simulink model "Simulation_with_controller"  (R2014b)
settings: Solver=ode45  StartTime=0.0  StopTime=T  RelTol=1e-3
undefined symbols (not defined in the file): a, L, ref, T, thetainit, Ts, xinit, yinit
settings Model: Creator=Oskar  LastModifiedBy=osklj59
settings OptimizationCC: UseDivisionForNetSlopeComputation=off  SimCompilerOptimization=off
settings DebuggingCC: UnderspecifiedInitializationDetection=Classic  MergeDetectMultiDrivingBlocksExec=none  FrameProcessingCompatibilityMsg=error  StateNameClashWarn=warning
settings RTWCC: RTWCompilerOptimization=off

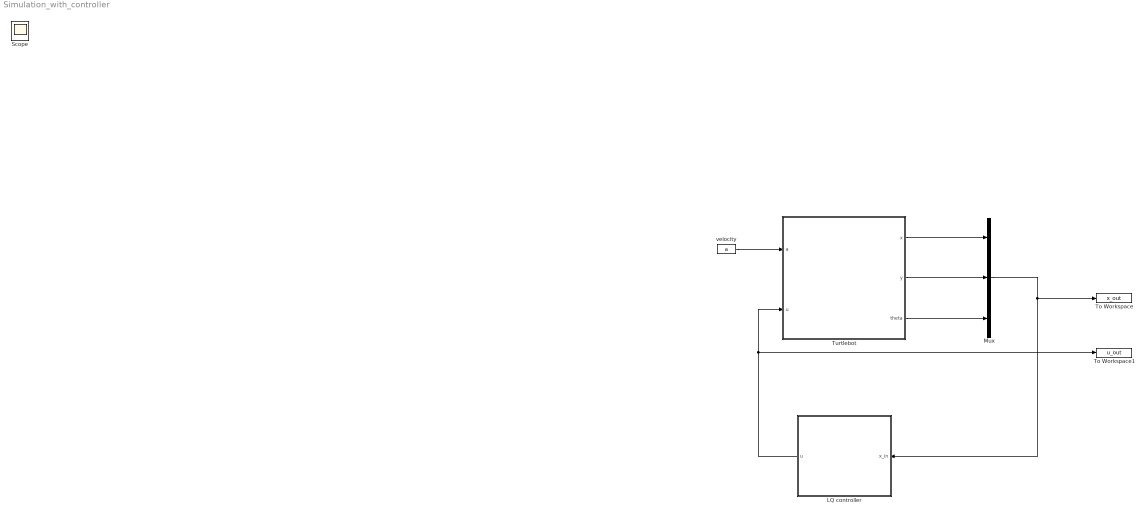
== system Simulation_with_controller ==
  LQ controller : Subsystem
  Mux : Mux  Inputs=3
  To Workspace : ToWorkspace  VariableName=x_out  SaveFormat=Timeseries  SampleTime=-1
  To Workspace1 : ToWorkspace  VariableName=u_out  SaveFormat=Timeseries  SampleTime=-1
  Turtlebot : Subsystem
  velocity : Constant  Value=a
  Scope : Scope
      settings: YMin=-0.4  YMax=0.8
  wires:
  Turtlebot/1("x ") -> Mux/1
  Mux/1 -> To Workspace/1, LQ controller/1(x_in)
  velocity/1 -> Turtlebot/1(a)
  Turtlebot/2("y ") -> Mux/2
  Turtlebot/3("theta ") -> Mux/3
  LQ controller/1(u) -> Turtlebot/2(u), To Workspace1/1

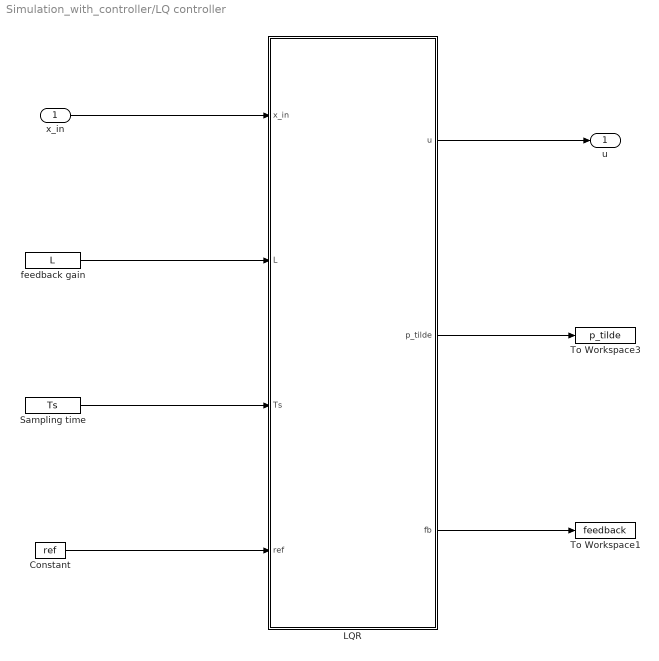
== system Simulation_with_controller/LQ controller ==
  x_in : Inport
  " LQR" : MATLAB Function
  Constant : Constant  Value=ref
  Sampling time : Constant  Value=Ts
  To Workspace1 : ToWorkspace  VariableName=feedback  SaveFormat=Timeseries  SampleTime=-1
  To Workspace3 : ToWorkspace  VariableName=p_tilde  SaveFormat=Timeseries  SampleTime=-1
  feedback gain : Constant  Value=L
  u : Outport
  wires:
  x_in/1 -> " LQR"/1(x_in)
  " LQR"/2(p_tilde) -> To Workspace3/1
  feedback gain/1 -> " LQR"/2(L)
  " LQR"/1(u) -> u/1
  Sampling time/1 -> " LQR"/3(Ts)
  Constant/1 -> " LQR"/4(ref)
  " LQR"/3(fb) -> To Workspace1/1

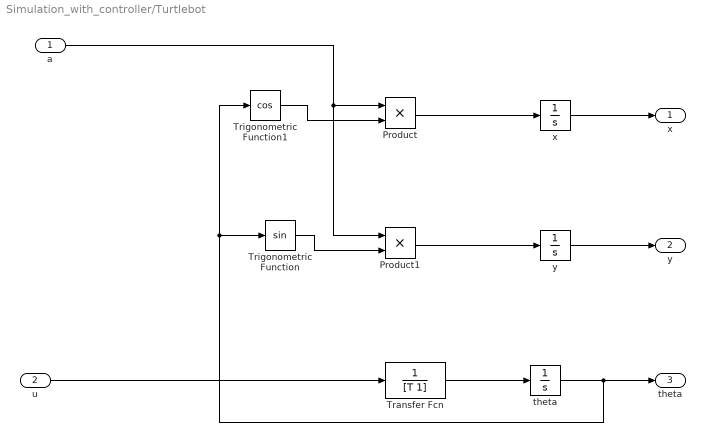
== system Simulation_with_controller/Turtlebot ==
  a : Inport
  u : Inport  Port=2
  Product : Product
  Product1 : Product
  Transfer Fcn : TransferFcn  Denominator=[T 1]
  Trigonometric Function : Trigonometry
  Trigonometric Function1 : Trigonometry  Operator=cos
  theta : Integrator  InitialCondition=thetainit
  x : Integrator  InitialCondition=xinit
  y : Integrator  InitialCondition=yinit
  "x " : Outport  PortDimensions=1
  "y " : Outport  Port=2
  "theta " : Outport  Port=3
  wires:
  a/1 -> Product1/1, Product/1
  x/1 -> "x "/1
  y/1 -> "y "/1
  theta/1 -> Trigonometric Function/1, Trigonometric Function1/1, "theta "/1
  u/1 -> Transfer Fcn/1
  Trigonometric Function1/1 -> Product/2
  Trigonometric Function/1 -> Product1/2
  Product/1 -> x/1
  Product1/1 -> y/1
  Transfer Fcn/1 -> theta/1

== matlab function Simulation_with_controller/LQ controller/ LQR ==
  data: u output; x_in input; p_tilde output; L input; Ts input; ref input; fb output
function [u, p_tilde,fb]  = LQ(x_in, L, Ts, ref)

persistent prev_index p_tilde_prev

if isempty(prev_index)
    prev_index = 1;
end

if isempty(p_tilde_prev)
    p_tilde_prev = [0 0]';
end

th_error_prev = p_tilde_prev(2);

x = x_in(1);
y = x_in(2);
theta = x_in(3);

%Find closest point to trajectory i.e find s(t)
[x_close,y_close,index,Max_index] = find_intersection_x_y(x, y, ref, prev_index);

%Check if outside trajectory
if(index>Max_index-1) 
    index = Max_index-1;
end

%find reference trajectory at S(t)
if(index > 1)
    xp=[x ; y]; 
    x1=[ref(index-1,1);ref(index-1,2)]; 
    x2=[ref(index+1,1);ref(index+1,2)];
    v=xp-x1; w=x2-x1;
    a = v'*w/(w'*w);

    theta0 = a*ref(index+1,3)+(1-a)*ref(index-1,3);
    u0 = a*ref(index+1,4)+(1-a)*ref(index-1,4);
else
    
    theta0 = ref(index,3);
    u0 = ref(index,4);
end

%Compute distance error
z =(y - y_close)*cos(theta0)-(x - x_close)*sin(theta0);

%Compute error heading
th_error = theta - theta0;

p_tilde = [z;th_error]; %acutal values

fb = L' * p_tilde;

u = u0 - fb;


prev_index = index;
p_tilde_prev = p_tilde;

end
